simulink subsystem "yj_ro"  (R2024b)
settings: Solver=VariableStepAuto  StartTime=0.0  StopTime=10.0  RelTol=1e-3
libraries: fl_lib x1, SimscapeFluids_lib x1
settings Model: Creator=degoede  LastModifiedBy=degoede

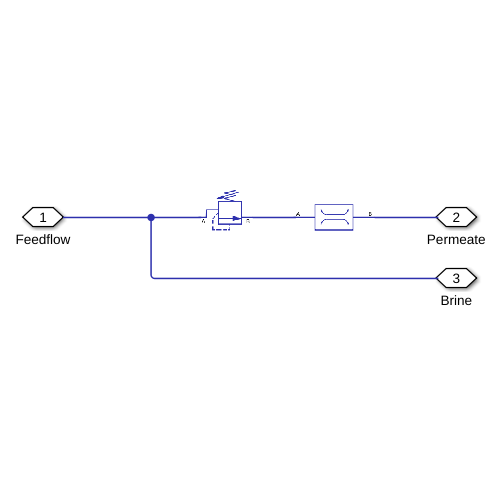
[thumbnail: Simulink's stored preview of the top-level diagram]
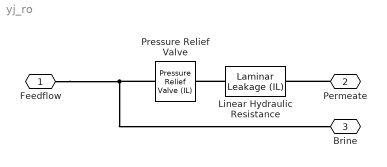
== system yj_ro ==
  Linear Hydraulic Resistance : fl_lib/Isothermal Liquid/Elements/Laminar Leakage (IL)  cross_section_geometry=6  diameter=1e-3 m  inner_diameter=5e-4 m  outer_diameter=1e-3 m  width=1e-3 m  height=0.1 m  major_axis=1e-3 m  minor_axis=5e-4 m  side_length=1e-3 m  length=5 m  resistance=mem_resist MPa*s/m^3
      settings: InternalSimscapePortConfiguration="{\"Bottom\":[],\"Left\":[{\"id\":\"A\",\"label\":\"A\",\"type\":\"foundation.isothermal_liquid.isothermal_liquid\"}],\"Right\":[{\"id\":\"B\",\"label\":\"B\",\"type\":\"foundation.isothermal_liquid.isothermal_liquid\"}],\"Top\":[]}"
  Pressure Relief Valve : SimscapeFluids_lib/Isothermal Liquid/Valves & Orifices/Pressure Control Valves/Pressure Relief Valve (IL)  set_pressure_spec=foundation.enum.constant_controlled.constant  opening_spec=1  pressure_spec=fluids.isothermal_liquid.valves_orifices.enum.pressure_control_spec.dp  p_set_gauge=0.1 MPa  p_set_differential=osmotic_pressure MPa  p_range=5e4 Pa  area_max=0.3 m^2  area_leak=1e-12 m^2  p_diff_TLU=[30.15e5 : 15e3 : 31.35e5] Pa  p_gauge_TLU=[0.2 : 0.2 : 1.2] MPa  valve_area_TLU=[1 : 1 : 9] .* 1e-5 m^2  vol_flow_TLU=[1e-09, 3.6e-05, 8.9e-05, .00015, .00023, .00031] m^3/s  area=inf m^2  Cd=0.7  Re_c=150  smoothing_factor=0  pressure_recovery=simscape.enum.onoff.off  opening_dynamics=0  tau=0.1 s
      settings: LibrarySourceBlock=SimscapeFluids_lib/Isothermal Liquid/Valves & Orifices/Pressure Control Valves/Pressure Relief Valve (IL)  InternalSimscapePortConfiguration="{\"Bottom\":[],\"Left\":[{\"id\":\"A\",\"label\":\"A\",\"type\":\"foundation.isothermal_liquid.isothermal_liquid\"}],\"Right\":[{\"id\":\"B\",\"label\":\"B\",\"type\":\"foundation.isothermal_liquid.isothermal_liquid\"}],\"Top\":[]}"
  Feedflow : PMIOPort  Side=Left
  Permeate : PMIOPort  Port=2  Side=Right
  Brine : PMIOPort  Port=3  Side=Right
  connections:
  Pressure Relief Valve/LConn1 -- Feedflow/RConn1 -- Brine/RConn1
  Linear Hydraulic Resistance/LConn1 -- Pressure Relief Valve/RConn1
  Permeate/RConn1 -- Linear Hydraulic Resistance/RConn1
